simulink model "Hysteresis"  (R2018b)
settings: Solver=VariableStepAuto  StartTime=0.0  StopTime=10.0  MaxStep=1/(100*fn)  MinStep=1/(1000*fn)  RelTol=1e-3
values from neighbouring files (symbols this model uses):
  A = sqrt(2/3)*[1 -0.5 -0.5; 0 sqrt(3)/2 -sqrt(3)/2; sqrt(0.5) sqrt(0.5) sqrt(0.5)]    [Comm_Vect.m]    (also in clarke_conc.m)
  Ai = inv(A)    [Comm_Vect.m]    (also in clarke_conc.m)
  delta = pi/2    (= 1.57079632679)    [clarke_conc.m]
  fv = 0.0033    [Comm_Vect.m]    (also in clarke_conc.m)
  J = 0.05    [Comm_Vect.m]    (also in clarke_conc.m)
  kp_i = 1    [clarke_conc.m]
  kp_v = 1    [clarke_conc.m]
  Ld = 0.245    [Comm_Vect.m]    (also in clarke_conc.m)
  Lq = 0.245    [Comm_Vect.m]    (also in clarke_conc.m)
  p = 60*fn/Nn    (= 2)    [Comm_Vect.m]    (also in clarke_conc.m)
  phi_f = 0.711    [Comm_Vect.m]    (also in clarke_conc.m)
  Rs = 10.5    [Comm_Vect.m]    (also in clarke_conc.m)
  Ti_v = J/fv    (= 15.1515151515)    [clarke_conc.m]
  ws = 2*pi*fn/p    (= 157.079632679)    [Comm_Vect.m]    (also in clarke_conc.m)
undefined symbols (not defined in the file or in its folder): jsin
settings Model: Creator=cindyiskandar  LastModifiedBy=cindyiskandar
settings SolverCC: ZeroCrossAlgorithm=Adaptive
settings DebuggingCC: IgnoredZcDiagnostic=none

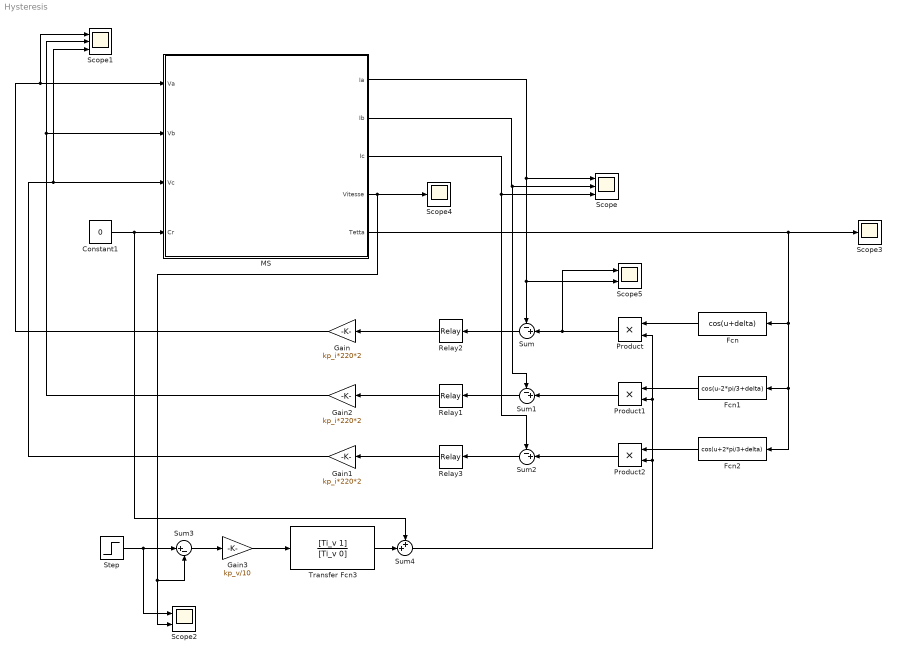
== system Hysteresis ==
  Constant1 : Constant  Value=0
  Fcn : Fcn  Expr=cos(u+delta)
  Fcn1 : Fcn  Expr=cos(u-2*pi/3+delta)
  Fcn2 : Fcn  Expr=cos(u+2*pi/3+delta)
  Gain : Gain  Gain=kp_i*220*2
  Gain1 : Gain  Gain=kp_i*220*2
  Gain2 : Gain  Gain=kp_i*220*2
  Gain3 : Gain  Gain=kp_v/10
  MS : Subsystem
  Product : Product
  Product1 : Product
  Product2 : Product
  Relay1 : Relay  OnSwitchValue=0.01  OffSwitchValue=-0.01  OffOutputValue=-1
  Relay2 : Relay  OnSwitchValue=0.01  OffSwitchValue=-0.01  OffOutputValue=-1
  Relay3 : Relay  OnSwitchValue=0.01  OffSwitchValue=-0.01  OffOutputValue=-1
  Scope : Scope  NumInputPorts=3
  Scope1 : Scope  NumInputPorts=3
  Scope2 : Scope  NumInputPorts=2
  Scope3 : Scope
  Scope4 : Scope
  Scope5 : Scope  NumInputPorts=2
  Step : Step  After=ws  SampleTime=0
  Sum : Sum  Inputs=-+|
  Sum1 : Sum  Inputs=-+|
  Sum2 : Sum  Inputs=-+|
  Sum3 : Sum  Inputs=|+-
  Sum4 : Sum  Inputs=++|
  Transfer Fcn3 : TransferFcn  Numerator=[Ti_v 1]  Denominator=[Ti_v 0]
  wires:
  MS/3(Ic) -> Scope/3, Sum2/1
  Constant1/1 -> Sum4/1, MS/4(Cr)
  MS/4(Vitesse) -> Scope2/2, Sum3/2, Scope4/1
  MS/5("Tetta ") -> Fcn2/1, Fcn1/1, Fcn/1, Scope3/1
  Gain3/1 -> Transfer Fcn3/1
  Relay2/1 -> Gain/1
  MS/2(Ib) -> Scope/2, Sum1/1
  Relay3/1 -> Gain1/1
  Step/1 -> Scope2/1, Sum3/1
  MS/1(Ia) -> Scope/1, Scope5/2, Sum/1
  Fcn1/1 -> Product1/1
  Transfer Fcn3/1 -> Sum4/2
  Sum3/1 -> Gain3/1
  Fcn2/1 -> Product2/1
  Relay1/1 -> Gain2/1
  Product1/1 -> Sum1/2
  Product/1 -> Scope5/1, Sum/2
  Fcn/1 -> Product/1
  Product2/1 -> Sum2/2
  Sum2/1 -> Relay3/1
  Sum1/1 -> Relay1/1
  Sum/1 -> Relay2/1
  Gain/1 -> MS/1(Va), Scope1/1
  Gain2/1 -> MS/2(Vb), Scope1/2
  Gain1/1 -> MS/3(Vc), Scope1/3
  Sum4/1 -> Product/2, Product1/2, Product2/2

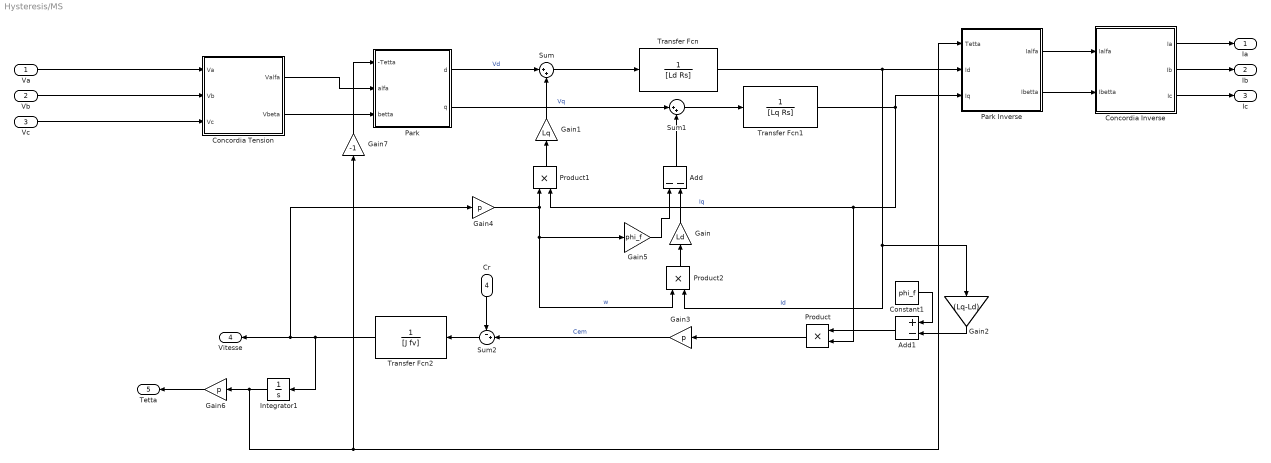
== system Hysteresis/MS ==
  Va : Inport
  Vb : Inport  Port=2
  Vc : Inport  Port=3
  Cr : Inport  Port=4
  Add : Sum  Inputs=--
  Add1 : Sum  Inputs=+-
  "Concordia Tension " : Subsystem
  "Concordia Inverse " : Subsystem
  Constant1 : Constant  Value=phi_f
  Gain : Gain  Gain=Ld
  Gain1 : Gain  Gain=Lq
  Gain2 : Gain  Gain=(Lq-Ld)
  Gain3 : Gain  Gain=p
  Gain4 : Gain  Gain=p
  Gain5 : Gain  Gain=phi_f
  Gain6 : Gain  Gain=p
  Gain7 : Gain  Gain=-1
  Integrator1 : Integrator  InitialCondition=ws
  Park : Subsystem
  Park Inverse : Subsystem
  Product : Product
  Product1 : Product
  Product2 : Product
  Sum : Sum  Inputs=|++
  Sum1 : Sum  Inputs=|++
  Sum2 : Sum  Inputs=-+|
  Transfer Fcn : TransferFcn  Denominator=[Ld Rs]
  Transfer Fcn1 : TransferFcn  Denominator=[Lq Rs]
  Transfer Fcn2 : TransferFcn  Denominator=[J fv]
  Ia : Outport
  Ib : Outport  Port=2
  Ic : Outport  Port=3
  Vitesse : Outport  Port=4
  "Tetta " : Outport  Port=5
  wires:
  Gain2/1 -> Add1/2
  Sum1/1 -> Transfer Fcn1/1
  Gain1/1 -> Sum/2
  Va/1 -> "Concordia Tension "/1("Va ")
  Gain/1 -> Add/2
  "Concordia Inverse "/2(Ib) -> Ib/1
  Vb/1 -> "Concordia Tension "/2("Vb ")
  Constant1/1 -> Add1/1
  Transfer Fcn1/1 -> Park Inverse/3("Iq "), Product1/2, Product/2  "Iq"
  "Concordia Inverse "/3(Ic) -> Ic/1
  Add1/1 -> Product/1
  Add/1 -> Sum1/2
  Park Inverse/2(Ibetta) -> "Concordia Inverse "/2(Ibetta)
  Park Inverse/1(Ialfa) -> "Concordia Inverse "/1(Ialfa)
  Sum/1 -> Transfer Fcn/1
  "Concordia Tension "/2("Vbeta ") -> Park/3("betta ")
  "Concordia Tension "/1(Valfa) -> Park/2(alfa)
  Vc/1 -> "Concordia Tension "/3(Vc)
  "Concordia Inverse "/1(Ia) -> Ia/1
  Park/1(d) -> Sum/1  "Vd"
  Transfer Fcn/1 -> Product2/2, Gain2/1, Park Inverse/2(Id)  "Id"
  Park/2(q) -> Sum1/1  "Vq"
  Product/1 -> Gain3/1
  Cr/1 -> Sum2/1
  Sum2/1 -> Transfer Fcn2/1
  Transfer Fcn2/1 -> Gain4/1, Vitesse/1, Integrator1/1
  Product1/1 -> Gain1/1
  Gain4/1 -> Product2/1, Gain5/1, Product1/1  "w"
  Product2/1 -> Gain/1
  Gain5/1 -> Add/1
  Gain6/1 -> "Tetta "/1
  Integrator1/1 -> Gain7/1, Park Inverse/1("Tetta "), Gain6/1
  Gain7/1 -> Park/1(-Tetta)
  Gain3/1 -> Sum2/2  "Cem"

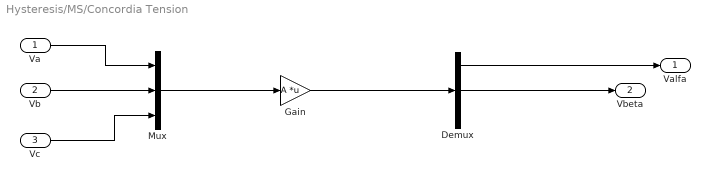
== system Hysteresis/MS/Concordia Tension  ==
  "Va " : Inport
  "Vb " : Inport  Port=2
  Vc : Inport  Port=3
  Demux : Demux  Outputs=3
  Gain : Gain  Gain=A  Multiplication=Matrix(K*u) (u vector)
  Mux : Mux  Inputs=3
  Valfa : Outport
  "Vbeta " : Outport  Port=2
  wires:
  Demux/1 -> Valfa/1
  "Va "/1 -> Mux/1
  Mux/1 -> Gain/1
  Gain/1 -> Demux/1
  "Vb "/1 -> Mux/2
  Vc/1 -> Mux/3
  Demux/2 -> "Vbeta "/1

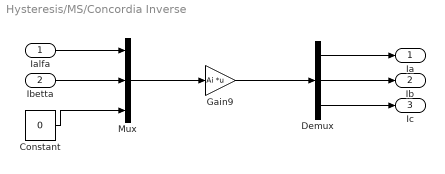
== system Hysteresis/MS/Concordia Inverse  ==
  Ialfa : Inport
  Ibetta : Inport  Port=2
  Constant : Constant  Value=0
  Demux : Demux  Outputs=3
  Gain9 : Gain  Gain=Ai  Multiplication=Matrix(K*u) (u vector)
  Mux : Mux  Inputs=3
  Ia : Outport
  Ib : Outport  Port=2
  Ic : Outport  Port=3
  wires:
  Demux/3 -> Ic/1
  Gain9/1 -> Demux/1
  Demux/1 -> Ia/1
  Demux/2 -> Ib/1
  Ibetta/1 -> Mux/2
  Ialfa/1 -> Mux/1
  Mux/1 -> Gain9/1
  Constant/1 -> Mux/3

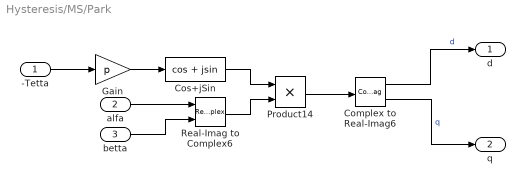
== system Hysteresis/MS/Park ==
  -Tetta : Inport
  alfa : Inport  Port=2
  "betta " : Inport  Port=3
  Complex to Real-Imag6 : ComplexToRealImag
  Cos+jSin : Trigonometry  Operator=cos + jsin
  Gain : Gain  Gain=p
  Product14 : Product
  Real-Imag to Complex6 : RealImagToComplex
  d : Outport
  q : Outport  Port=2
  wires:
  alfa/1 -> Real-Imag to Complex6/1
  Product14/1 -> Complex to Real-Imag6/1
  "betta "/1 -> Real-Imag to Complex6/2
  Complex to Real-Imag6/1 -> d/1  "d"
  Complex to Real-Imag6/2 -> q/1  "q"
  Real-Imag to Complex6/1 -> Product14/2
  Cos+jSin/1 -> Product14/1
  Gain/1 -> Cos+jSin/1
  -Tetta/1 -> Gain/1

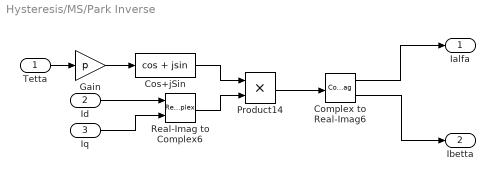
== system Hysteresis/MS/Park Inverse ==
  "Tetta " : Inport
  Id : Inport  Port=2
  "Iq " : Inport  Port=3
  Complex to Real-Imag6 : ComplexToRealImag
  Cos+jSin : Trigonometry  Operator=cos + jsin
  Gain : Gain  Gain=p
  Product14 : Product
  Real-Imag to Complex6 : RealImagToComplex
  Ialfa : Outport
  Ibetta : Outport  Port=2
  wires:
  Id/1 -> Real-Imag to Complex6/1
  Product14/1 -> Complex to Real-Imag6/1
  "Iq "/1 -> Real-Imag to Complex6/2
  Complex to Real-Imag6/1 -> Ialfa/1
  Complex to Real-Imag6/2 -> Ibetta/1
  Real-Imag to Complex6/1 -> Product14/2
  Cos+jSin/1 -> Product14/1
  Gain/1 -> Cos+jSin/1
  "Tetta "/1 -> Gain/1
